simulink model "PI_Controlled_SAPF_dq_theory"  (R2023a)
settings: Solver=VariableStepAuto  StartTime=0.0  StopTime=2  RelTol=1e-3
libraries: spsThreePhaseVIMeasurementLib x3, dspfdesign x2, spsSeriesRLCBranchLib x2, spsUniversalBridgeLib x2, slpidlib x1, spsThreePhaseSeriesRLCBranchLib x1, spsThreePhaseSourceLib x1, spsVoltageMeasurementLib x1, spspowerguiLib x1
settings Model: Creator=Nitiz Khanal  LastModifiedBy=Nitiz Khanal
settings DataIOCC: ReturnWorkspaceOutputs=off

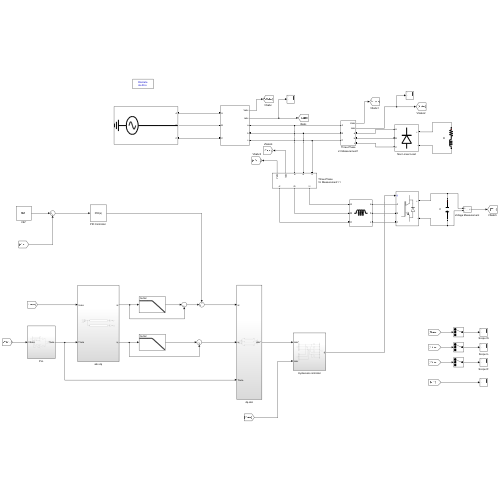
[thumbnail: Simulink's stored preview of the top-level diagram]
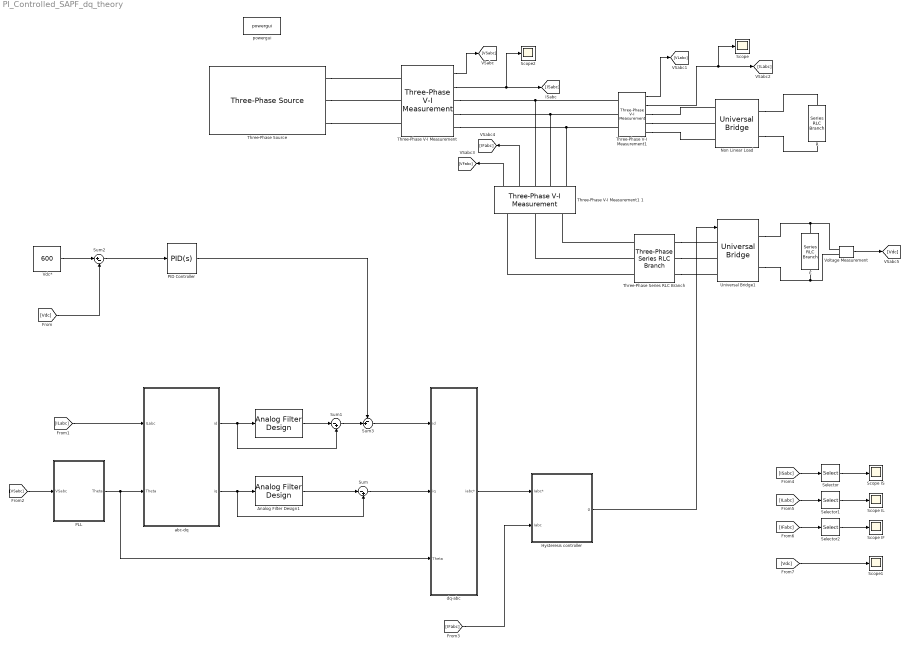
== system PI_Controlled_SAPF_dq_theory ==
  "     " : dspfdesign/Analog Filter Design  method=Butterworth  filttype=Lowpass  N=8  Wlo=10*pi  Whi=80  Rp=2  Rs=40
  Analog Filter Design1 : dspfdesign/Analog Filter Design  method=Butterworth  filttype=Lowpass  N=8  Wlo=10*pi  Whi=80  Rp=2  Rs=40
  C : spsSeriesRLCBranchLib/Series RLC Branch  LConnTagsString=__new0  RConnTagsString=__new0  BranchType=C  Resistance=1  Inductance=1e-3  SetiL0=off  InitialCurrent=0  Capacitance=1500e-6  Setx0=on  InitialVoltage=500  Measurements=None
  Hysteresis controller : Subsystem
  Non Linear Load : spsUniversalBridgeLib/Universal Bridge  Arms=3  SnubberResistance=1e5  SnubberCapacitance=inf  Device=Diodes  Ron=1e-3  Lon=0  ForwardVoltages="[  0  0  ]"  ForwardVoltage=0  GTOparameters=[ 10e-6 , 20e-6 ]  IGBTparameters=[ 1e-6 , 2e-6 ]  Measurements=None  Measurements_2=None  converterType=Rectifier
  "PID Controller " : slpidlib/PID Controller  Controller=PID  Form=Parallel  TimeDomain=Continuous-time  UseExternalTs=off  SampleTime=-1  IntegratorMethod=Forward Euler  FilterMethod=Forward Euler  ControllerParametersSource=internal  P=1.5  I=50  UseKiTs=off  D=0  N=100  UseFilter=on  TunerSelectOption=Transfer Function Based (PID Tuner App)  InitialConditionSource=internal  InitialConditionForIntegrator=0  InitialConditionForFilter=0  DifferentiatorICPrevScaledInput=0  ExternalReset=none  TrackingMode=off  Kt=1  LimitOutput=off  SatLimitsSource=internal  UpperSaturationLimit=inf  LowerSaturationLimit=-inf  LinearizeAsGain=on  AntiWindupMode=none  Kb=1  LimitIntegrator=off  UpperIntegratorSaturationLimit=inf  LowerIntegratorSaturationLimit=-inf  POutMin=[]  POutMax=[]  IOutMin=[]  IOutMax=[]  DOutMin=[]  DOutMax=[]  NOutMin=[]  NOutMax=[]  SumOutMin=[]  SumOutMax=[]  SaturationOutMin=[]  SaturationOutMax=[]  PParamMin=[]  PParamMax=[]  IParamMin=[]  IParamMax=[]  DParamMin=[]  DParamMax=[]  NParamMin=[]  NParamMax=[]  KbParamMin=[]  KbParamMax=[]  KtParamMin=[]  KtParamMax=[]  KbOutMin=[]  KbOutMax=[]  KtOutMin=[]  KtOutMax=[]  IntegratorOutMin=[]  IntegratorOutMax=[]  FilterOutMin=[]  FilterOutMax=[]  SumI1OutMin=[]  SumI1OutMax=[]  SumI2OutMin=[]  SumI2OutMax=[]  SumI3OutMin=[]  SumI3OutMax=[]  SumI4OutMin=[]  SumI4OutMax=[]  SumDOutMin=[]  SumDOutMax=[]  DifferentiatorOutMin=[]  DifferentiatorOutMax=[]  FilterDiffOutCoefMin=[]  FilterDiffOutCoefMax=[]  ReciprocalOutMin=[]  ReciprocalOutMax=[]  SumDenOutMin=[]  SumDenOutMax=[]  SumNumOutMin=[]  SumNumOutMax=[]  DivideOutMin=[]  DivideOutMax=[]  UdiffTsProdOutMin=[]  UdiffTsProdOutMax=[]  NTsProdOutMin=[]  NTsProdOutMax=[]  UintegralTsProdOutMin=[]  UintegralTsProdOutMax=[]  UngainTsProdOutMin=[]  UngainTsProdOutMax=[]  ClampingZeroOutDataTypeStr=Inherit: Inherit via back propagation  ClampingZeroOutMin=[]  ClampingZeroOutMax=[]  FilterDenConstantOutDataTypeStr=Inherit: Inherit via back propagation  FilterDenConstantOutMin=[]  FilterDenConstantOutMax=[]  PCopyOutDataTypeStr=Inherit: Inherit via back propagation  PCopyOutMin=[]  PCopyOutMax=[]  NCopyOutDataTypeStr=Inherit: Inherit via back propagation  NCopyOutMin=[]  NCopyOutMax=[]  IntegratorContinuousStateAttributes=''  IntegratorStateMustResolveToSignalObject=off  IntegratorRTWStateStorageClass=Auto  FilterContinuousStateAttributes=''  FilterStateMustResolveToSignalObject=off  FilterRTWStateStorageClass=Auto  ParallelPVariant=InternalParameters  IdealPVariant=Disabled  IVariant=InternalParameters  DVariant=InternalParameters  IntegratorVariant=Continuous  SatVariant=Disabled  AWVariant=Passthrough  PCopyVariant=Disabled  TRVariant=Disabled  FdbkBlocksVariant=Forward  IdealPFdbkVariant=Disabled  SatFdbkVariant=Disabled  DerivativeFilterVariant=ContFilter  NVariant=InternalParameters  NCopyVariant=Disabled  FilterICVariant=InternalICsFilter  IntegratorICVariant=InternalICs  ExternalResetVariant=Disabled  TRSumVariant=Passthrough  SumFdbkVariant=Disabled  SumVariant=Sum_PID  TsampFilterVariant=InternalTs  TsampNgainVariant=Passthrough  TsampIntegralVariant=Disabled_SignalSpec  ExternalSaturationOutDataTypeStr=Inherit: Same as second input
  PLL : Subsystem
  R : spsSeriesRLCBranchLib/Series RLC Branch  LConnTagsString=__new0  RConnTagsString=__new0  BranchType=RL  Resistance=30  Inductance=100e-3  SetiL0=off  InitialCurrent=0  Capacitance=1e-6  Setx0=off  InitialVoltage=0  Measurements=None
  Scope : Scope
  Scope IF : Scope
  Scope IL : Scope
  Scope IS : Scope
  Scope1 : Scope
  Scope2 : Scope
  Selector : Selector  InputPortWidth=3  IndexOptions=Index vector (dialog)  Indices=1  OutputSizes=1
  Selector1 : Selector  InputPortWidth=3  IndexOptions=Index vector (dialog)  Indices=1  OutputSizes=1
  Selector2 : Selector  InputPortWidth=3  IndexOptions=Index vector (dialog)  Indices=1  OutputSizes=1
  Sum : Sum  Inputs=|-+
  Sum1 : Sum  Inputs=|-+
  Sum2 : Sum  Inputs=|+-
  Sum3 : Sum  Inputs=-+|
  Three-Phase Series RLC Branch : spsThreePhaseSeriesRLCBranchLib/Three-Phase Series RLC Branch  LConnTagsString=A|B|C  RConnTagsString=A|B|C  BranchType=L  Resistance=1  Inductance=2e-3  Capacitance=1e-6  Measurements=None
  Three-Phase V-I Measurement : spsThreePhaseVIMeasurementLib/Three-Phase V-I Measurement  VoltageMeasurement=phase-to-ground  SetLabelV=off  LabelV=Vabc  Vpu=off  VpuLL=off  CurrentMeasurement=yes  SetLabelI=off  LabelI=Iabc  Ipu=off  Pbase=100e6  Vbase=500e3  OutputType=Complex  PhasorSimulation=off  PSBequivalent=0
  "Three-Phase V-I Measurement1 " : spsThreePhaseVIMeasurementLib/Three-Phase V-I Measurement  VoltageMeasurement=phase-to-ground  SetLabelV=off  LabelV=Vabc  Vpu=off  VpuLL=off  CurrentMeasurement=yes  SetLabelI=off  LabelI=Iabc  Ipu=off  Pbase=100e6  Vbase=500e3  OutputType=Complex  PhasorSimulation=off  PSBequivalent=0
  Three-Phase V-I Measurement1 1 : spsThreePhaseVIMeasurementLib/Three-Phase V-I Measurement  VoltageMeasurement=phase-to-ground  SetLabelV=off  LabelV=Vabc  Vpu=off  VpuLL=off  CurrentMeasurement=yes  SetLabelI=off  LabelI=Iabc  Ipu=off  Pbase=100e6  Vbase=500e3  OutputType=Complex  PhasorSimulation=off  PSBequivalent=0
  Three-Phase Source : spsThreePhaseSourceLib/Three-Phase Source  InternalConnection=Yg  VoltagePhases=off  Voltage=220  PhaseAngle=0  Voltage_phases=[25e3 25e3 25e3]/sqrt(3)  PhaseAngles_phases=[0 -120 +120]  Frequency=50  NonIdealSource=off  SpecifyImpedance=off  Resistance=0.8929  Inductance=16.58e-3  ShortCircuitLevel=100e6  BaseVoltage=25e3  XRratio=7  BusType=swing  Pref=10e3  Qref=0  Prefabc=[10e3, 10e3, 10e3]  Qrefabc=[0, 0, 0]  Qmin=-inf  Qmax=inf
  Universal Bridge1 : spsUniversalBridgeLib/Universal Bridge  Arms=3  SnubberResistance=1e5  SnubberCapacitance=inf  Device=IGBT / Diodes  Ron=1e-3  Lon=0  ForwardVoltages="[  0  0  ]"  ForwardVoltage=0  GTOparameters=[ 10e-6 , 20e-6 ]  IGBTparameters=[ 1e-6 , 2e-6 ]  Measurements=None  Measurements_2=None  converterType=Rectifier
  Vdc* : Constant  Value=600
  "Voltage Measurement " : spsVoltageMeasurementLib/Voltage Measurement  PhasorSimulation=off  OutputType=Complex  PSBequivalent=0
  abc-dq : Subsystem
  dq-abc : Subsystem
  powergui : spspowerguiLib/powergui  Priority=1  SimulationMode=Discrete  SampleTime=2e-6  frequency=60  Iterations=50  frequencyindice=50  Pbase=100e6  ErrMax=1e-4  UnitsV=kV  UnitsW=MW  buscounter=0  FunctionMessages=off  echomessages=off  EnableUseOfTLC=off  CurrentSourceSwitches=off  DisableSnubberDevices=off  DisableRonSwitches=off  DisableVfSwitches=off  DisplayEquations=off  AutomaticDiscreteSolvers=off  SolverType=Tustin/Backward Euler (TBE)  Interpol=off  ExternalGateDelay=off  methode=off  Ts=100  x0status=blocks  SPID=on  SwTol=0  HookPort=off  NonlinearTolerance=1e-4  nMaxIteration=100  ContinueOnMaxIteration=off  RestoreLinks=warning  ResistiveCurrentMeasurement=off  Frange=[0:2:500]  Ylog=off  Xlog=on  ShowGrid=off  save=off  variable=ZData  structure=0  ZoomFFT=off  StartTime=0.0  cycles=1  DisplayStyle=1  fundamental=60  FreqAxis=off  MaxFrequency=1000  frequencyindicesteady=1  RmsSteady=1  display=off
  wires:
  Three-Phase V-I Measurement/1 -> [VSabc]
  Three-Phase V-I Measurement/2 -> Scope2/1, [ISabc]
  "Three-Phase V-I Measurement1 "/1 -> [VLabc]
  "Three-Phase V-I Measurement1 "/2 -> Scope/1, [ILabc]
  Three-Phase V-I Measurement1 1/1 -> [VFabc]
  Three-Phase V-I Measurement1 1/2 -> [IFabc]
  "Voltage Measurement "/1 -> [Vdc]
  PLL/1(Theta) -> dq-abc/3(Theta), abc-dq/2(Theta)
  abc-dq/1(id) -> Sum1/2, "     "/1
  abc-dq/2(iq) -> Analog Filter Design1/1, Sum/2
  Analog Filter Design1/1 -> Sum/1
  "     "/1 -> Sum1/1
  Sum2/1 -> "PID Controller "/1
  Vdc*/1 -> Sum2/1
  Sum/1 -> dq-abc/2(iq)
  dq-abc/1(iabc*) -> Hysteresis controller/1(Iabc*)
  [Vdc] -> Sum2/2
  [ILabc] -> abc-dq/1(ILabc)
  [VSabc] -> PLL/1(VSabc)
  Hysteresis controller/1(g) -> Universal Bridge1/1
  [IFabc] -> Hysteresis controller/2(Iabc)
  Selector/1 -> Scope IS/1
  Selector1/1 -> Scope IL/1
  Selector2/1 -> Scope IF/1
  [ILabc] -> Selector1/1
  [IFabc] -> Selector2/1
  [Vdc] -> Scope1/1
  [ISabc] -> Selector/1
  Sum1/1 -> Sum3/2
  Sum3/1 -> dq-abc/1(id)
  "PID Controller "/1 -> Sum3/1
  connections:
  Three-Phase Source/RConn1 -- Three-Phase V-I Measurement/LConn1
  Three-Phase Source/RConn2 -- Three-Phase V-I Measurement/LConn2
  Three-Phase Source/RConn3 -- Three-Phase V-I Measurement/LConn3
  Three-Phase V-I Measurement/RConn1 -- Three-Phase V-I Measurement1 1/RConn1 -- "Three-Phase V-I Measurement1 "/LConn1
  Three-Phase V-I Measurement/RConn2 -- "Three-Phase V-I Measurement1 "/LConn2 -- Three-Phase V-I Measurement1 1/RConn2
  Three-Phase V-I Measurement/RConn3 -- "Three-Phase V-I Measurement1 "/LConn3 -- Three-Phase V-I Measurement1 1/RConn3
  "Three-Phase V-I Measurement1 "/RConn1 -- Non Linear Load/LConn1
  "Three-Phase V-I Measurement1 "/RConn2 -- Non Linear Load/LConn2
  "Three-Phase V-I Measurement1 "/RConn3 -- Non Linear Load/LConn3
  Non Linear Load/RConn1 -- R/LConn1
  Non Linear Load/RConn2 -- R/RConn1
  Three-Phase Series RLC Branch/RConn1 -- Universal Bridge1/LConn1
  Three-Phase Series RLC Branch/RConn2 -- Universal Bridge1/LConn2
  Three-Phase Series RLC Branch/RConn3 -- Universal Bridge1/LConn3
  Three-Phase Series RLC Branch/LConn1 -- Three-Phase V-I Measurement1 1/LConn3
  Three-Phase Series RLC Branch/LConn2 -- Three-Phase V-I Measurement1 1/LConn2
  Three-Phase Series RLC Branch/LConn3 -- Three-Phase V-I Measurement1 1/LConn1
  Universal Bridge1/RConn1 -- "Voltage Measurement "/LConn1 -- C/LConn1
  Universal Bridge1/RConn2 -- "Voltage Measurement "/LConn2 -- C/RConn1

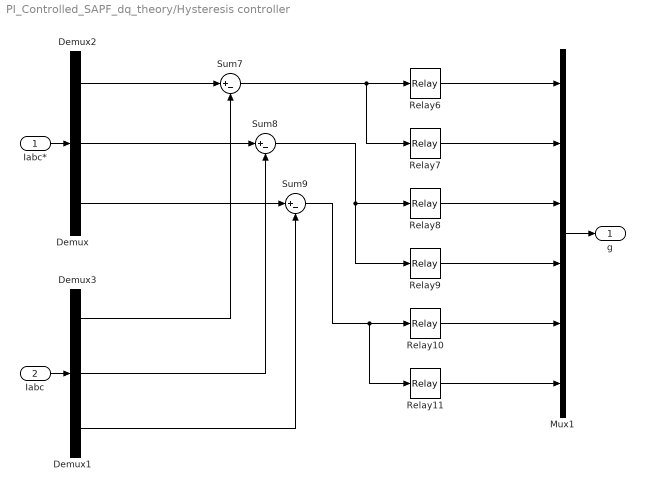
== system PI_Controlled_SAPF_dq_theory/Hysteresis controller ==
  Iabc* : Inport
  Iabc : Inport  Port=2
  Demux{,1..3} (4 alike) : Demux  Outputs=3
  Mux1 : Mux  Inputs=6
  Relay10 : Relay  OnSwitchValue=0.001  OffSwitchValue=-0.01
  Relay11 : Relay  OnSwitchValue=0.001  OffSwitchValue=-0.01  OnOutputValue=0  OffOutputValue=1
  Relay6 : Relay  OnSwitchValue=0.001  OffSwitchValue=-0.01
  Relay7 : Relay  OnSwitchValue=0.001  OffSwitchValue=-0.01  OnOutputValue=0  OffOutputValue=1
  Relay8 : Relay  OnSwitchValue=0.001  OffSwitchValue=-0.01
  Relay9 : Relay  OnSwitchValue=0.001  OffSwitchValue=-0.01  OnOutputValue=0  OffOutputValue=1
  Sum7 : Sum  Inputs=|+-
  Sum8 : Sum  Inputs=|+-
  Sum9 : Sum  Inputs=|+-
  g : Outport
  wires:
  Iabc/1 -> Demux1/1
  Sum7/1 -> Relay7/1, Relay6/1
  Relay7/1 -> Mux1/2
  Sum9/1 -> Relay11/1, Relay10/1
  Iabc*/1 -> Demux/1
  Relay10/1 -> Mux1/5
  Relay6/1 -> Mux1/1
  Sum8/1 -> Relay9/1, Relay8/1
  Demux2/3 -> Sum9/1
  Relay8/1 -> Mux1/3
  Relay9/1 -> Mux1/4
  Relay11/1 -> Mux1/6
  Demux3/3 -> Sum9/2
  Demux3/2 -> Sum8/2
  Demux3/1 -> Sum7/2
  Demux2/1 -> Sum7/1
  Demux2/2 -> Sum8/1
  Mux1/1 -> g/1

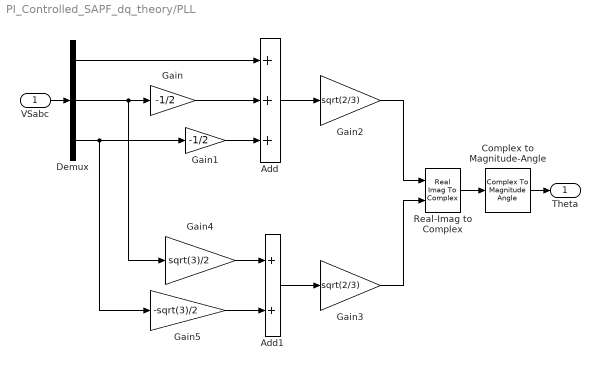
== system PI_Controlled_SAPF_dq_theory/PLL ==
  VSabc : Inport
  Add : Sum  Inputs=+++
  Add1 : Sum
  Complex to Magnitude-Angle : ComplexToMagnitudeAngle  Output=Angle
  Demux : Demux  Outputs=3
  Gain : Gain  Gain=-1/2
  Gain1 : Gain  Gain=-1/2
  Gain2 : Gain  Gain=sqrt(2/3)
  Gain3 : Gain  Gain=sqrt(2/3)
  Gain4 : Gain  Gain=sqrt(3)/2
  Gain5 : Gain  Gain=-sqrt(3)/2
  Real-Imag to Complex : RealImagToComplex
  Theta : Outport
  wires:
  Demux/3 -> Gain5/1, Gain1/1
  Add1/1 -> Gain3/1
  Gain/1 -> Add/2
  Real-Imag to Complex/1 -> Complex to Magnitude-Angle/1
  Gain2/1 -> Real-Imag to Complex/1
  Gain1/1 -> Add/3
  Demux/2 -> Gain4/1, Gain/1
  VSabc/1 -> Demux/1
  Demux/1 -> Add/1
  Gain5/1 -> Add1/2
  Gain3/1 -> Real-Imag to Complex/2
  Gain4/1 -> Add1/1
  Add/1 -> Gain2/1
  Complex to Magnitude-Angle/1 -> Theta/1

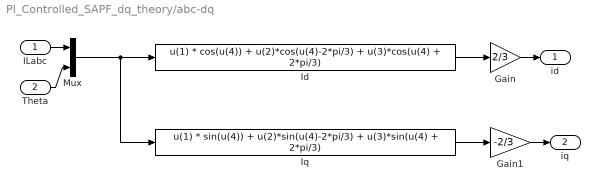
== system PI_Controlled_SAPF_dq_theory/abc-dq ==
  ILabc : Inport
  Theta : Inport  Port=2
  Gain : Gain  Gain=2/3
  Gain1 : Gain  Gain=-2/3
  Id : Fcn  Expr=u(1) * cos(u(4)) + u(2)*cos(u(4)-2*pi/3) + u(3)*cos(u(4) + 2*pi/3)
  Iq : Fcn  Expr=u(1) * sin(u(4)) + u(2)*sin(u(4)-2*pi/3) + u(3)*sin(u(4) + 2*pi/3)
  Mux : Mux  Inputs=2
  id : Outport
  iq : Outport  Port=2
  wires:
  Mux/1 -> Iq/1, Id/1
  Id/1 -> Gain/1
  ILabc/1 -> Mux/1
  Iq/1 -> Gain1/1
  Gain/1 -> id/1
  Gain1/1 -> iq/1
  Theta/1 -> Mux/2

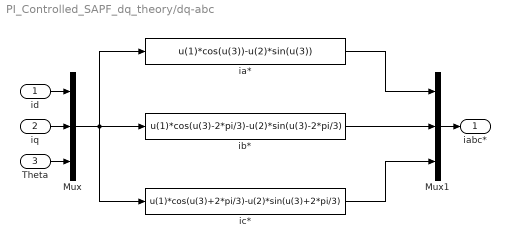
== system PI_Controlled_SAPF_dq_theory/dq-abc ==
  id : Inport
  iq : Inport  Port=2
  Theta : Inport  Port=3
  Mux : Mux  Inputs=3
  Mux1 : Mux  Inputs=3
  ia* : Fcn  Expr=u(1)*cos(u(3))-u(2)*sin(u(3))
  ib* : Fcn  Expr=u(1)*cos(u(3)-2*pi/3)-u(2)*sin(u(3)-2*pi/3)
  ic* : Fcn  Expr=u(1)*cos(u(3)+2*pi/3)-u(2)*sin(u(3)+2*pi/3)
  iabc* : Outport
  wires:
  Mux1/1 -> iabc*/1
  Theta/1 -> Mux/3
  Mux/1 -> ic*/1, ia*/1, ib*/1
  ic*/1 -> Mux1/3
  ib*/1 -> Mux1/2
  ia*/1 -> Mux1/1
  iq/1 -> Mux/2
  id/1 -> Mux/1
